simulink model "montecarloSim"  (R2017a)
settings: Solver=FixedStepDiscrete  StartTime=0.0  StopTime=inf  FixedStep=1  RelTol=1e-3
undefined symbols (not defined in the file or in its folder): MAXITER, tol
libraries: simulink x3
settings Model: Creator=Enrico Donato  LastModifiedBy=Enrico Donato

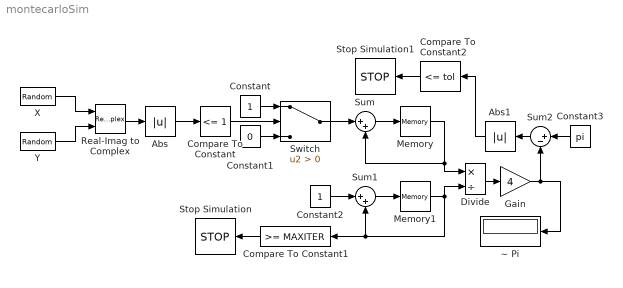
== system montecarloSim ==
  Abs : Abs
  Abs1 : Abs
  Compare To Constant : simulink/Logic and Bit Operations/Compare To Constant  relop=<=  const=1  OutDataTypeStr=boolean
  Compare To Constant1 : simulink/Logic and Bit Operations/Compare To Constant  relop=>=  const=MAXITER  OutDataTypeStr=boolean
  Compare To Constant2 : simulink/Logic and Bit Operations/Compare To Constant  relop=<=  const=tol  OutDataTypeStr=boolean
  Constant : Constant
  Constant1 : Constant  Value=0
  Constant2 : Constant
  Constant3 : Constant  Value=pi
  Divide : Product  Inputs=*/
  Gain : Gain  Gain=4
  Memory : Memory
  Memory1 : Memory  X0=1
  Real-Imag to Complex : RealImagToComplex
  Stop Simulation : Stop
  Stop Simulation1 : Stop
  Sum : Sum  Inputs=|++
  Sum1 : Sum  Inputs=|++
  Sum2 : Sum  Inputs=|+-
  Switch : Switch  Criteria=u2 > Threshold
  X : UniformRandomNumber  SampleTime=1
  Y : UniformRandomNumber  Seed=3  SampleTime=1
  ~ Pi : Display
      settings: Decimation=4
  wires:
  Y/1 -> Real-Imag to Complex/2
  X/1 -> Real-Imag to Complex/1
  Real-Imag to Complex/1 -> Abs/1
  Abs/1 -> Compare To Constant/1
  Compare To Constant/1 -> Switch/2
  Constant/1 -> Switch/1
  Constant1/1 -> Switch/3
  Switch/1 -> Sum/1
  Sum/1 -> Memory/1
  Memory/1 -> Divide/1, Sum/2
  Memory1/1 -> Divide/2, Sum1/2, Compare To Constant1/1
  Sum1/1 -> Memory1/1
  Constant2/1 -> Sum1/1
  Divide/1 -> Gain/1
  Gain/1 -> ~ Pi/1, Sum2/2
  Compare To Constant1/1 -> Stop Simulation/1
  Compare To Constant2/1 -> Stop Simulation1/1
  Constant3/1 -> Sum2/1
  Abs1/1 -> Compare To Constant2/1
  Sum2/1 -> Abs1/1
